simulink model "Home_5_4"  (R2016b)
settings: Solver=VariableStepAuto  StartTime=0.0  StopTime=runtime  RelTol=1e-3
values from neighbouring files (symbols this model uses):
  Isx_lim = 120    [Home54_init.m]
  Isy_lim = 120    [Home54_init.m]
  J = 0.05    [Ex5_2_init.m]    (also in Ex5_3_init.m; Home54_init.m = 0.5; homepart51.m)
  Ki_l = 8000    [Home54_init.m]
  Ki_w = 24000    [Home54_init.m]
  Kp_l = 2300    [Home54_init.m]
  Kp_w = 320    [Home54_init.m]
  L0 = 1e-4    (= 0.0001)    [Home54_init.m]
  L_s = 0.085    [Ex5_2_init.m]    (also in Ex5_3_init.m; Home54_init.m)
  L_set = 0.816    [Home54_init.m]
  Llim = 100    [Home54_init.m]
  p = 1    [Ex5_2_init.m]    (also in Ex5_3_init.m; Home54_init.m; homepart51.m)
  R_R = 0.2792    [Home54_init.m]
  rho0 = 1e-4    (= 0.0001)    [Home54_init.m]
  sigma = 1 - M^2/(L_s*L_r)    (= 0.0693425605536)    [Ex5_2_init.m]    (also in Ex5_3_init.m = 0.0693; Home54_init.m = 0.0693; homepart51.m)
  tau_r = 0.283    [Ex5_3_init.m]    (also in Home54_init.m)
  tau_u = 0.0005    [Home54_init.m]
  Tl = 10    [Home54_init.m]
  Wlim = 100    [Home54_init.m]
  Wm0 = 0    [Home54_init.m]
  Wm_set = 0.1    [Home54_init.m]
settings Model: Creator=Niels  LastModifiedBy=Niels

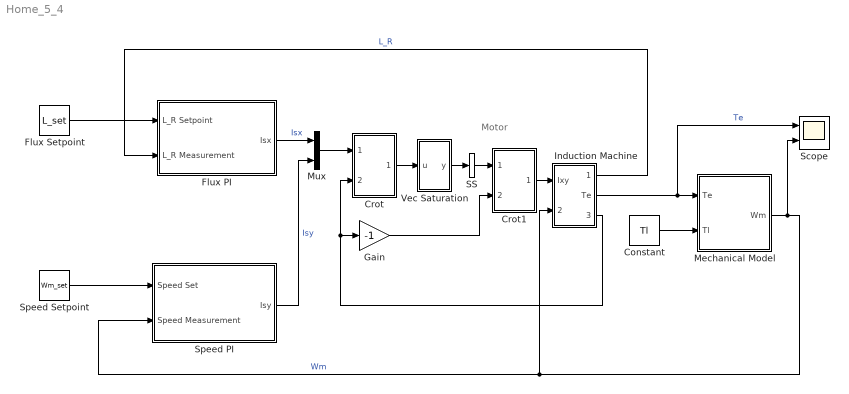
== system Home_5_4 ==
  note: Motor
  Constant : Constant  Value=Tl
  Crot : Subsystem
  Crot1 : Subsystem
  Flux PI : Subsystem
  Flux Setpoint : Constant  Value=L_set
  Gain : Gain  Gain=-1
  Induction Machine : Subsystem
  Mechanical Model : Subsystem
  Mux : Mux  Inputs=2
  SS : SignalSpecification  Dimensions=[2 1]
  Scope : Scope  NumInputPorts=2
  Speed PI : Subsystem
  "Speed Setpoint " : Constant  Value=Wm_set
  Vec Saturation : MATLAB Function  TreatAsAtomicUnit=on
  wires:
  Mechanical Model/1(Wm) -> Scope/2, Speed PI/2(Speed Measurement), Induction Machine/2(Wm)  "Wm"
  Induction Machine/2(Te) -> Scope/1, Mechanical Model/1(Te)  "Te"
  Flux Setpoint/1 -> Flux PI/1(L_R Setpoint)
  Induction Machine/1(L_R) -> Flux PI/2(L_R Measurement)  "L_R"
  Flux PI/1(Isx) -> Mux/1  "Isx"
  "Speed Setpoint "/1 -> Speed PI/1(Speed Set)
  Speed PI/1(Isy) -> Mux/2  "Isy"
  Constant/1 -> Mechanical Model/2(Tl)
  Mux/1 -> Crot/1(Isxy)
  Induction Machine/3(rho) -> Gain/1, Crot/2(rho)
  Crot/1(Ialpbet) -> Vec Saturation/1(u)
  Crot1/1(Isxy) -> Induction Machine/1(Ixy)
  Gain/1 -> Crot1/2(-rho)
  Vec Saturation/1(y) -> SS/1
  SS/1 -> Crot1/1(Ialphbet)

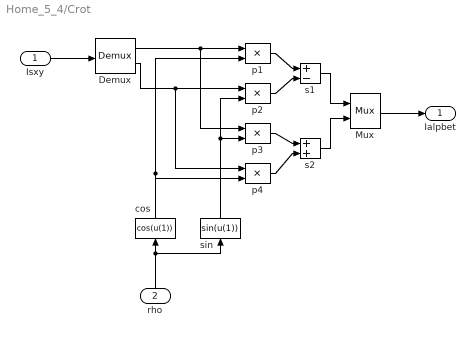
== system Home_5_4/Crot ==
  Isxy : Inport
  rho : Inport  Port=2
  Demux : Demux  Outputs=2
  Mux : Mux  Inputs=2
  cos : Fcn  Expr=cos(u(1))
  p{1..4} (4 alike) : Product  SaturateOnIntegerOverflow=on  RndMeth=Zero  InputSameDT=on  OutDataTypeStr=Inherit: Same as first input
  s1 : Sum  Inputs=+-  SaturateOnIntegerOverflow=on  InputSameDT=on  OutDataTypeStr=Inherit: Same as first input
  s2 : Sum  SaturateOnIntegerOverflow=on  InputSameDT=on  OutDataTypeStr=Inherit: Same as first input
  sin : Fcn  Expr=sin(u(1))
  Ialpbet : Outport
  wires:
  sin/1 -> p2/2, p3/2
  cos/1 -> p1/2, p4/2
  rho/1 -> cos/1, sin/1
  Isxy/1 -> Demux/1
  p2/1 -> s1/2
  s1/1 -> Mux/1
  Demux/1 -> p1/1, p3/1
  Mux/1 -> Ialpbet/1
  Demux/2 -> p2/1, p4/1
  s2/1 -> Mux/2
  p3/1 -> s2/1
  p1/1 -> s1/1
  p4/1 -> s2/2

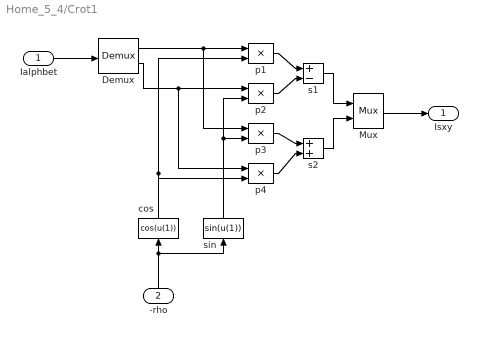
== system Home_5_4/Crot1 ==
  Ialphbet : Inport
  -rho : Inport  Port=2
  Demux : Demux  Outputs=2
  Mux : Mux  Inputs=2
  cos : Fcn  Expr=cos(u(1))
  p{1..4} (4 alike) : Product  SaturateOnIntegerOverflow=on  RndMeth=Zero  InputSameDT=on  OutDataTypeStr=Inherit: Same as first input
  s1 : Sum  Inputs=+-  SaturateOnIntegerOverflow=on  InputSameDT=on  OutDataTypeStr=Inherit: Same as first input
  s2 : Sum  SaturateOnIntegerOverflow=on  InputSameDT=on  OutDataTypeStr=Inherit: Same as first input
  sin : Fcn  Expr=sin(u(1))
  Isxy : Outport
  wires:
  sin/1 -> p2/2, p3/2
  cos/1 -> p1/2, p4/2
  -rho/1 -> cos/1, sin/1
  Ialphbet/1 -> Demux/1
  p2/1 -> s1/2
  s1/1 -> Mux/1
  Demux/1 -> p1/1, p3/1
  Mux/1 -> Isxy/1
  Demux/2 -> p2/1, p4/1
  s2/1 -> Mux/2
  p3/1 -> s2/1
  p1/1 -> s1/1
  p4/1 -> s2/2

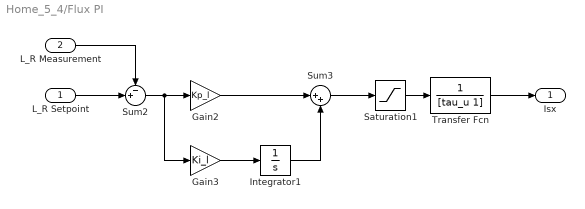
== system Home_5_4/Flux PI ==
  L_R Setpoint : Inport
  L_R Measurement : Inport  Port=2
  Gain2 : Gain  Gain=Kp_l
  Gain3 : Gain  Gain=Ki_l
  Integrator1 : Integrator  LimitOutput=on  UpperSaturationLimit=Llim  LowerSaturationLimit=-Llim
  Saturation1 : Saturate  UpperLimit=Isx_lim  LowerLimit=-Isx_lim
  Sum2 : Sum  Inputs=-+|
  Sum3 : Sum  Inputs=|++
  Transfer Fcn : TransferFcn  Denominator=[tau_u 1]
  Isx : Outport
  wires:
  Sum2/1 -> Gain3/1, Gain2/1
  Gain2/1 -> Sum3/1
  Integrator1/1 -> Sum3/2
  Gain3/1 -> Integrator1/1
  Sum3/1 -> Saturation1/1
  L_R Setpoint/1 -> Sum2/2
  L_R Measurement/1 -> Sum2/1
  Transfer Fcn/1 -> Isx/1
  Saturation1/1 -> Transfer Fcn/1

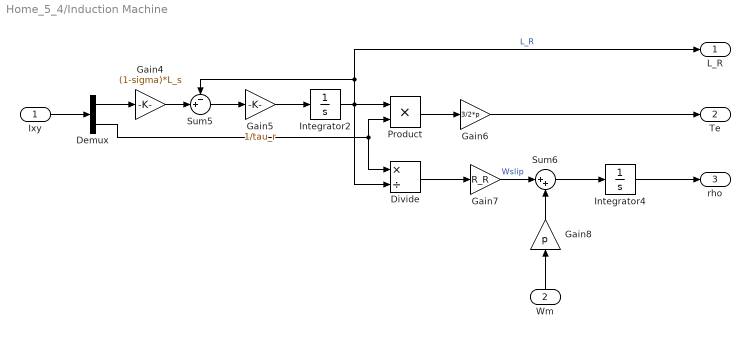
== system Home_5_4/Induction Machine ==
  Ixy : Inport
  Wm : Inport  Port=2
  Demux : Demux  Outputs=2
  Divide : Product  Inputs=*/
  Gain4 : Gain  Gain=(1-sigma)*L_s
  Gain5 : Gain  Gain=1/tau_r
  Gain6 : Gain  Gain=3/2*p
  Gain7 : Gain  Gain=R_R
  Gain8 : Gain  Gain=p
  Integrator2 : Integrator  InitialCondition=L0
  Integrator4 : Integrator  InitialCondition=rho0
  Product : Product
  Sum5 : Sum  Inputs=-+|
  Sum6 : Sum  Inputs=|++
  L_R : Outport
  Te : Outport  Port=2
  rho : Outport  Port=3
  wires:
  Gain5/1 -> Integrator2/1
  Gain4/1 -> Sum5/2
  Sum6/1 -> Integrator4/1
  Sum5/1 -> Gain5/1
  Demux/2 -> Divide/1, Product/2
  Gain6/1 -> Te/1
  Demux/1 -> Gain4/1
  Ixy/1 -> Demux/1
  Integrator2/1 -> Divide/2, Product/1, L_R/1, Sum5/1  "L_R"
  Divide/1 -> Gain7/1
  Gain8/1 -> Sum6/2
  Wm/1 -> Gain8/1
  Gain7/1 -> Sum6/1  "Wslip"
  Product/1 -> Gain6/1
  Integrator4/1 -> rho/1

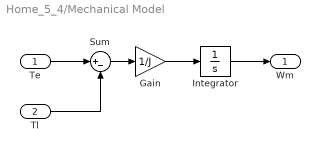
== system Home_5_4/Mechanical Model ==
  Te : Inport
  Tl : Inport  Port=2
  Gain : Gain  Gain=1/J
  Integrator : Integrator  InitialCondition=Wm0
  Sum : Sum  Inputs=|+-
  Wm : Outport
  wires:
  Te/1 -> Sum/1
  Tl/1 -> Sum/2
  Gain/1 -> Integrator/1
  Sum/1 -> Gain/1
  Integrator/1 -> Wm/1

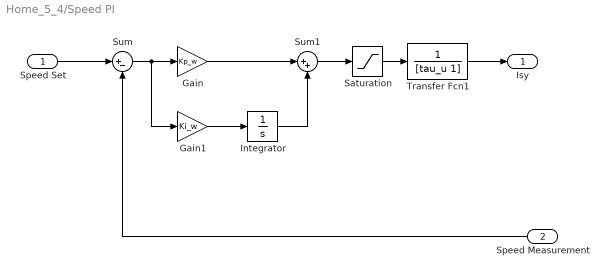
== system Home_5_4/Speed PI ==
  Speed Set : Inport
  Speed Measurement : Inport  Port=2
  Gain : Gain  Gain=Kp_w
  Gain1 : Gain  Gain=Ki_w
  Integrator : Integrator  LimitOutput=on  UpperSaturationLimit=Wlim  LowerSaturationLimit=-Wlim
  Saturation : Saturate  UpperLimit=Isy_lim  LowerLimit=-Isy_lim
  Sum : Sum  Inputs=|+-
  Sum1 : Sum  Inputs=|++
  Transfer Fcn1 : TransferFcn  Denominator=[tau_u 1]
  Isy : Outport
  wires:
  Integrator/1 -> Sum1/2
  Saturation/1 -> Transfer Fcn1/1
  Transfer Fcn1/1 -> Isy/1
  Speed Measurement/1 -> Sum/2
  Sum1/1 -> Saturation/1
  Sum/1 -> Gain1/1, Gain/1
  Speed Set/1 -> Sum/1
  Gain1/1 -> Integrator/1
  Gain/1 -> Sum1/1

== matlab function Home_5_4/Vec Saturation ==
  data: u input; y output; Imax parameter
function y = fcn(u,Imax)
y = u;
if u(1) >= Imax
    u(1) = Imax;
elseif u(1) <= -Imax
    u(1) = Imax;
end
if u(2) >= Imax
    u(2) = Imax;
elseif u(2) <= -Imax
    u(2) = Imax;
end
